simulink model "Copy_of_s_hover"  (Simulink 8.8)
settings: Solver=ode14x  StartTime=0.0  StopTime=inf  FixedStep=0.005  RelTol=1e-3  EnableMultiTasking=on
values from neighbouring files (symbols this model uses):
  b0_p = value    (= 0.1035)    [Copy_of_setup_lab_hover.m]
  b0_r = value    (= 0.1035)    [Copy_of_setup_lab_hover.m]
  b0_y = 0.0105    [Copy_of_setup_lab_hover.m]
  con = inv(con)    [Copy_of_setup_lab_hover.m]
  K_AMP = 3    [Copy_of_setup_lab_hover.m]    (also in setup_lab_hover.m; setup_lab_hover1.m)
  kd_p = 2 * wc_p    (= 23.3333333333)    [Copy_of_setup_lab_hover.m]
  kd_r = 2 * wc_r    (= 23.3333333333)    [Copy_of_setup_lab_hover.m]
  kd_y = 2 * wc_y    (= 8)    [Copy_of_setup_lab_hover.m]
  kp_p = wc_p ^ 2    (= 136.111111111)    [Copy_of_setup_lab_hover.m]
  kp_r = wc_r ^ 2    (= 136.111111111)    [Copy_of_setup_lab_hover.m]
  kp_y = wc_y ^ 2    (= 16)    [Copy_of_setup_lab_hover.m]
  VMAX_AMP = 24    [Copy_of_setup_lab_hover.m]    (also in setup_lab_hover.m; setup_lab_hover1.m)
  VMAX_DAC = 10    [Copy_of_setup_lab_hover.m]    (also in setup_lab_hover.m; setup_lab_hover1.m)
  w0_p = 35    [Copy_of_setup_lab_hover.m]
  w0_r = 35    [Copy_of_setup_lab_hover.m]
  w0_y = 28    [Copy_of_setup_lab_hover.m]
  wcf = 2 * pi * 20    (= 125.663706144)    [Copy_of_setup_lab_hover.m]    (also in setup_lab_hover.m; setup_lab_hover1.m)
  zetaf = 0.6    [Copy_of_setup_lab_hover.m]    (also in setup_lab_hover.m; setup_lab_hover1.m)
undefined symbols (not defined in the file or in its folder): A, B, C, D
libraries: simulink_extras x7, instrumentlib x2, aerolibanimutils x1
settings Model: LogicAnalyzerSignalOrdering=04bcc7a1-ed51-4d67-9ebe-09d7c85a2b61  SuppressorTable=22 serialization::archive 11 0 3 0 0 0 0 0  Creator=hpineros  LastModifiedBy=ronan  ExtModeTrigDuration=10000
settings SolverCC: PositivePriorityOrder=on
settings OptimizationCC: ExpressionDepthLimit=2147483647  InitFltsAndDblsToZero=on
settings DebuggingCC: SaveWithParameterizedLinksMsg=none  SolverPrmCheckMsg=warning
settings RTWCC: SystemTargetFile=quarc_windows.tlc  TemplateMakefile=quarc_default_tmf  Description=QuaRC Win32 Target
settings STFCustomTargetCC: TargetFcnLib=ansi_tfl_tmw.mat  TargetPreCompLibLocation=C:\PROGRA~3\QUARC\lib\2012b\windows\release  GeneratePreprocessorConditionals=Disable all  CPPClassGenCompliant=on  SystemTargetFile=quarc_windows.tlc
settings GRTTargetCC: TargetFcnLib=ansi_tfl_tmw.mat  TargetPreCompLibLocation=C:\PROGRA~3\QUARC\lib\2012b\windows\release  ParMdlRefBuildCompliant=off  CompOptLevelCompliant=off  ConcurrentExecutionCompliant=off  MatFileLogging=off  UseToolchainInfoCompliant=off  ExtMode=on  ExtModeMexFile=quarc_comm

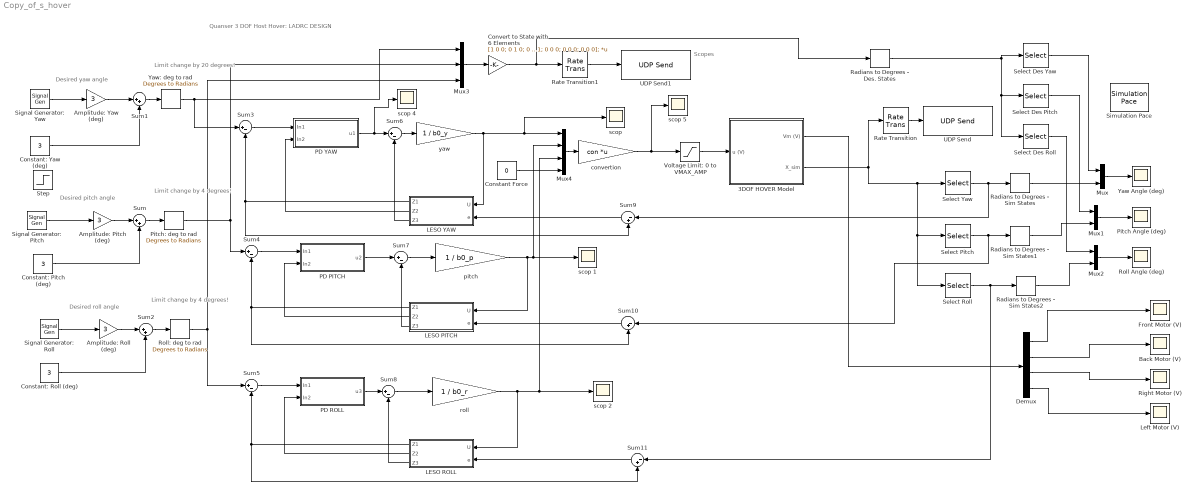
== system Copy_of_s_hover ==
  note: Quanser 3 DOF Host Hover:
      | LADRC DESIGN
  note: Scopes
  note: Limit change by
      | 4 degrees!
  note: Limit change by
      | 20 degrees!
  note: Limit change by
      | 4 degrees!
  note: Desired roll angle
  note: Desired pitch angle
  note: Desired yaw angle
  3DOF HOVER Model : Subsystem
  Amplitude: Pitch (deg) : Gain  Gain=3
  Amplitude: Roll (deg) : Gain  Gain=3
  Amplitude: Yaw (deg) : Gain  Gain=3
  Back Motor (V) : Scope
  Constant Force : Constant  Value=0
  Constant: Pitch (deg) : Constant  Value=3
  Constant: Roll (deg) : Constant  Value=3
  Constant: Yaw (deg) : Constant  Value=3
  Convert to State with 6 Elements : Gain  Gain=[1 0 0; 0 1 0; 0 0 1; 0 0 0; 0 0 0; 0 0 0];  Multiplication=Matrix(K*u)
  Demux : Demux
  Front Motor (V) : Scope
  LESO PITCH : Subsystem
  LESO ROLL : Subsystem
  LESO YAW : Subsystem
  Left Motor (V) : Scope
  Mux : Mux  Inputs=2
  Mux1 : Mux  Inputs=2
  Mux2 : Mux  Inputs=2
  Mux3 : Mux  Inputs=3
  Mux4 : Mux
  PD PITCH : Subsystem
  PD ROLL : Subsystem
  PD YAW : Subsystem
  Pitch Angle (deg) : Scope
  Pitch: deg to rad : simulink_extras/Transformations/Degrees to Radians
  Radians to Degrees - Des. States : simulink_extras/Transformations/Radians to Degrees
  Radians to Degrees - Sim States : simulink_extras/Transformations/Radians to Degrees
  Radians to Degrees - Sim States1 : simulink_extras/Transformations/Radians to Degrees
  Radians to Degrees - Sim States2 : simulink_extras/Transformations/Radians to Degrees
  Rate Transition : RateTransition  OutPortSampleTime=0.005
  Rate Transition1 : RateTransition  OutPortSampleTime=0.005
  Right Motor (V) : Scope
  Roll Angle (deg) : Scope
  Roll: deg to rad : simulink_extras/Transformations/Degrees to Radians
  Select Des Pitch : Selector  InputPortWidth=6  IndexOptions=Index vector (dialog)  Indices=2  OutputSizes=1
  Select Des Roll : Selector  InputPortWidth=6  IndexOptions=Index vector (dialog)  Indices=3  OutputSizes=1
  Select Des Yaw : Selector  InputPortWidth=6  IndexOptions=Index vector (dialog)  Indices=1  OutputSizes=1
  Select Pitch : Selector  InputPortWidth=6  IndexOptions=Index vector (dialog)  Indices=2  OutputSizes=1
  Select Roll : Selector  InputPortWidth=6  IndexOptions=Index vector (dialog)  Indices=3  OutputSizes=1
  Select Yaw : Selector  InputPortWidth=6  IndexOptions=Index vector (dialog)  Indices=1  OutputSizes=1
  Signal Generator: Pitch : SignalGenerator  WaveForm=square  Frequency=0.1
  Signal Generator: Roll : SignalGenerator  WaveForm=square  Frequency=0.08
  Signal Generator: Yaw : SignalGenerator  WaveForm=square  Frequency=0.04
  Simulation Pace : aerolibanimutils/Simulation Pace  SimulationPace=1  SleepMode=MATLAB Thread  OutputPaceError=off  SampleTime=0.01
  Step : Step  Time=0  SampleTime=0
  Sum : Sum  Inputs=|++
  Sum1 : Sum  Inputs=|++
  Sum10 : Sum  Inputs=|-+
  Sum11 : Sum  Inputs=|-+
  Sum2 : Sum  Inputs=|++
  Sum{3..8} (6 alike) : Sum  Inputs=|+-
  Sum9 : Sum  Inputs=|-+
  UDP Send : instrumentlib/UDP Send  Host=localhost  Port=9092  LocalPort=9091  EnableBlockingMode=on  ByteOrder=BigEndian
  UDP Send1 : instrumentlib/UDP Send  Host=localhost  Port=9094  LocalPort=9093  EnableBlockingMode=on  ByteOrder=BigEndian
  Voltage Limit: 0 to VMAX_AMP : Saturate  UpperLimit=VMAX_AMP  LowerLimit=0
  Yaw Angle (deg) : Scope
  Yaw: deg to rad : simulink_extras/Transformations/Degrees to Radians
  convertion : Gain  Gain=con  Multiplication=Matrix(K*u)  SaturateOnIntegerOverflow=on  OutDataTypeStr=Inherit: Same as input  ParamDataTypeStr=Inherit: Same as input
  pitch : Gain  Gain=1 / b0_p  SaturateOnIntegerOverflow=on  OutDataTypeStr=Inherit: Same as input  ParamDataTypeStr=Inherit: Same as input
  roll : Gain  Gain=1 / b0_r  SaturateOnIntegerOverflow=on  OutDataTypeStr=Inherit: Same as input  ParamDataTypeStr=Inherit: Same as input
  scop {,1..2,4..5} (5 alike) : Scope
  yaw : Gain  Gain=1 / b0_y  SaturateOnIntegerOverflow=on  OutDataTypeStr=Inherit: Same as input  ParamDataTypeStr=Inherit: Same as input
  wires:
  3DOF HOVER Model/1(Vm (V)) -> Demux/1
  Select Des Roll/1 -> Mux2/1
  Select Des Pitch/1 -> Mux1/1
  Select Des Yaw/1 -> Mux/1
  Radians to Degrees - Des. States/1 -> Select Des Yaw/1, Select Des Roll/1, Select Des Pitch/1
  Select Roll/1 -> Sum11/1, Radians to Degrees - Sim States2/1
  Select Pitch/1 -> Sum10/1, Radians to Degrees - Sim States1/1
  Select Yaw/1 -> Sum9/1, Radians to Degrees - Sim States/1
  Mux2/1 -> Roll Angle (deg)/1
  3DOF HOVER Model/2(X_sim) -> Select Yaw/1, Select Pitch/1, Select Roll/1, Rate Transition/1
  Mux1/1 -> Pitch Angle (deg)/1
  Mux/1 -> Yaw Angle (deg)/1
  Demux/1 -> Front Motor (V)/1
  Demux/2 -> Back Motor (V)/1
  Demux/3 -> Right Motor (V)/1
  Demux/4 -> Left Motor (V)/1
  Rate Transition/1 -> UDP Send/1
  Rate Transition1/1 -> UDP Send1/1
  Roll: deg to rad/1 -> Mux3/3, Sum5/1
  Pitch: deg to rad/1 -> Sum4/1, Mux3/2
  Yaw: deg to rad/1 -> Sum3/1, Mux3/1
  Sum2/1 -> Roll: deg to rad/1
  Amplitude: Roll (deg)/1 -> Sum2/1
  Constant: Roll (deg)/1 -> Sum2/2
  Sum/1 -> Pitch: deg to rad/1
  Amplitude: Pitch (deg)/1 -> Sum/1
  Constant: Pitch (deg)/1 -> Sum/2
  Sum1/1 -> Yaw: deg to rad/1
  Amplitude: Yaw (deg)/1 -> Sum1/1
  Constant: Yaw (deg)/1 -> Sum1/2
  Mux3/1 -> Convert to State with 6 Elements/1
  Convert to State with 6 Elements/1 -> Radians to Degrees - Des. States/1, Rate Transition1/1
  Sum3/1 -> PD YAW/1(In1)
  LESO YAW/1(Z1) -> Sum9/2, Sum3/2
  LESO PITCH/1(Z1) -> Sum10/2, Sum4/2
  LESO ROLL/1(Z1) -> Sum5/2, Sum11/2
  Sum5/1 -> PD ROLL/1(In1)
  Sum4/1 -> PD PITCH/1(In1)
  LESO YAW/2(Z2) -> PD YAW/2(In2)
  LESO PITCH/2(Z2) -> PD PITCH/2(In2)
  LESO ROLL/2(Z2) -> PD ROLL/2(In2)
  PD YAW/1(u1) -> scop 4/1, Sum6/1
  LESO YAW/3(Z3) -> Sum6/2
  PD PITCH/1(u2) -> Sum7/1
  LESO PITCH/3(Z3) -> Sum7/2
  PD ROLL/1(u3) -> Sum8/1
  LESO ROLL/3(Z3) -> Sum8/2
  Sum6/1 -> yaw/1
  yaw/1 -> LESO YAW/1(U), "scop "/1, Mux4/1
  Sum7/1 -> pitch/1
  Sum8/1 -> roll/1
  pitch/1 -> Mux4/2, scop 1/1, LESO PITCH/1(U)
  roll/1 -> scop 2/1, Mux4/3, LESO ROLL/1(U)
  Sum9/1 -> LESO YAW/2(e)
  Sum10/1 -> LESO PITCH/2(e)
  Sum11/1 -> LESO ROLL/2(e)
  convertion/1 -> Voltage Limit: 0 to VMAX_AMP/1, scop 5/1
  Mux4/1 -> convertion/1
  Constant Force/1 -> Mux4/4
  Voltage Limit: 0 to VMAX_AMP/1 -> 3DOF HOVER Model/1(u (V))
  Radians to Degrees - Sim States/1 -> Mux/2
  Radians to Degrees - Sim States1/1 -> Mux1/2
  Radians to Degrees - Sim States2/1 -> Mux2/2
  Signal Generator: Roll/1 -> Amplitude: Roll (deg)/1
  Signal Generator: Pitch/1 -> Amplitude: Pitch (deg)/1
  Signal Generator: Yaw/1 -> Amplitude: Yaw (deg)/1

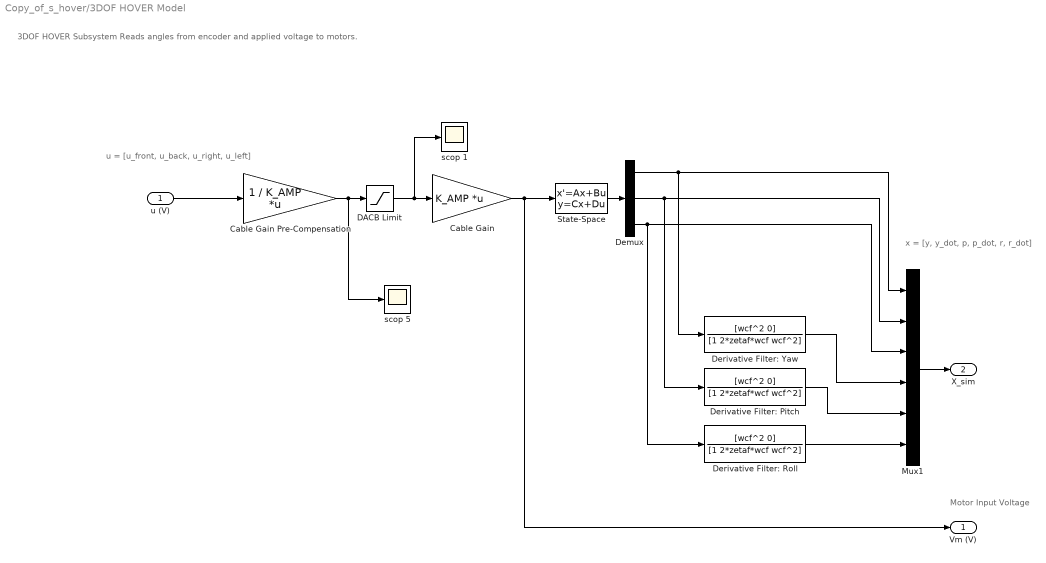
== system Copy_of_s_hover/3DOF HOVER Model ==
  note: 3DOF HOVER Subsystem
      | Reads angles from encoder and applied voltage to motors.
  note: Motor Input Voltage
  note: u = [u_front, u_back, u_right, u_left]
  note: x = [y, y_dot, p, p_dot, r, r_dot]
  u (V) : Inport
  Cable Gain : Gain  Gain=K_AMP  Multiplication=Matrix(K*u)  SaturateOnIntegerOverflow=on  OutDataTypeStr=Inherit: Same as input  ParamDataTypeStr=Inherit: Same as input
  Cable Gain Pre-Compensation : Gain  Gain=1 / K_AMP  Multiplication=Matrix(K*u)  SaturateOnIntegerOverflow=on  OutDataTypeStr=Inherit: Same as input  ParamDataTypeStr=Inherit: Same as input
  DACB Limit : Saturate  UpperLimit=VMAX_DAC  LowerLimit=-VMAX_DAC
  Demux : Demux  Outputs=3
  Derivative Filter: Pitch : TransferFcn  Numerator=[wcf^2 0]  Denominator=[1 2*zetaf*wcf wcf^2]
  Derivative Filter: Roll : TransferFcn  Numerator=[wcf^2 0]  Denominator=[1 2*zetaf*wcf wcf^2]
  Derivative Filter: Yaw : TransferFcn  Numerator=[wcf^2 0]  Denominator=[1 2*zetaf*wcf wcf^2]
  Mux1 : Mux  Inputs=6
  State-Space : StateSpace  A=A  B=B  C=C  D=D  X0=0
  scop 1 : Scope
  scop 5 : Scope
  Vm (V) : Outport
  X_sim : Outport  Port=2
  wires:
  Demux/3 -> Derivative Filter: Roll/1, Mux1/3
  Demux/2 -> Derivative Filter: Pitch/1, Mux1/2
  Derivative Filter: Roll/1 -> Mux1/6
  Derivative Filter: Pitch/1 -> Mux1/5
  Derivative Filter: Yaw/1 -> Mux1/4
  Demux/1 -> Derivative Filter: Yaw/1, Mux1/1
  State-Space/1 -> Demux/1
  Mux1/1 -> X_sim/1
  Cable Gain/1 -> State-Space/1, Vm (V)/1
  DACB Limit/1 -> scop 1/1, Cable Gain/1
  Cable Gain Pre-Compensation/1 -> scop 5/1, DACB Limit/1
  u (V)/1 -> Cable Gain Pre-Compensation/1

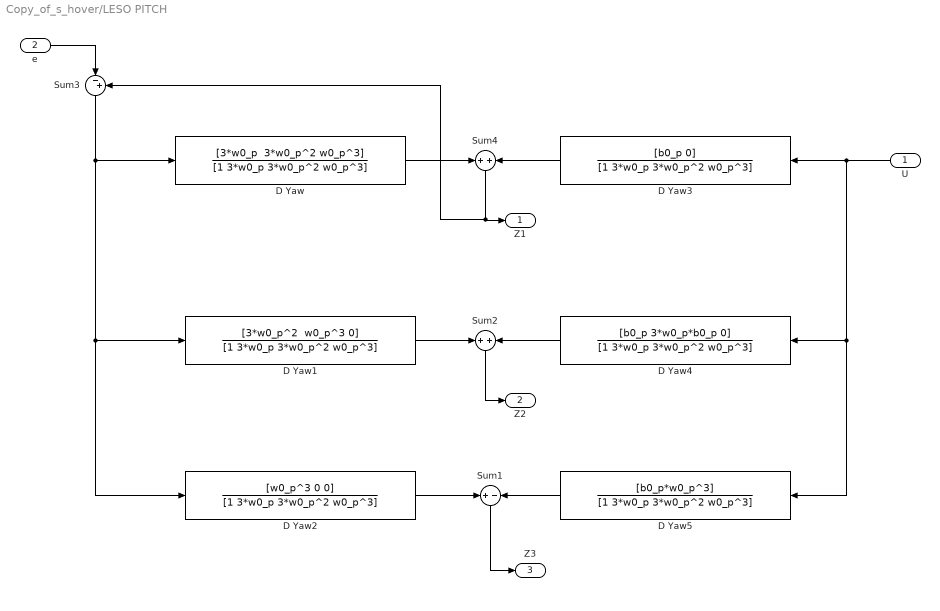
== system Copy_of_s_hover/LESO PITCH ==
  U : Inport
  e : Inport  Port=2
  D Yaw : TransferFcn  Numerator="[3*w0_p  3*w0_p^2 w0_p^3]"  Denominator=[1 3*w0_p 3*w0_p^2 w0_p^3]
  D Yaw1 : TransferFcn  Numerator="[3*w0_p^2  w0_p^3 0]"  Denominator=[1 3*w0_p 3*w0_p^2 w0_p^3]
  D Yaw2 : TransferFcn  Numerator=[w0_p^3 0 0]  Denominator=[1 3*w0_p 3*w0_p^2 w0_p^3]
  D Yaw3 : TransferFcn  Numerator=[b0_p 0]  Denominator=[1 3*w0_p 3*w0_p^2 w0_p^3]
  D Yaw4 : TransferFcn  Numerator=[b0_p 3*w0_p*b0_p 0]  Denominator=[1 3*w0_p 3*w0_p^2 w0_p^3]
  D Yaw5 : TransferFcn  Numerator=[b0_p*w0_p^3]  Denominator=[1 3*w0_p 3*w0_p^2 w0_p^3]
  Sum1 : Sum  Inputs=+|-
  Sum2 : Sum  Inputs=+|+
  Sum3 : Sum  Inputs=|-+
  Sum4 : Sum  Inputs=+|+
  Z1 : Outport
  Z2 : Outport  Port=2
  Z3 : Outport  Port=3
  wires:
  e/1 -> Sum3/1
  Sum3/1 -> D Yaw2/1, D Yaw1/1, D Yaw/1
  U/1 -> D Yaw5/1, D Yaw4/1, D Yaw3/1
  D Yaw2/1 -> Sum1/1
  D Yaw5/1 -> Sum1/2
  Sum1/1 -> Z3/1
  D Yaw1/1 -> Sum2/1
  D Yaw4/1 -> Sum2/2
  Sum2/1 -> Z2/1
  D Yaw/1 -> Sum4/1
  D Yaw3/1 -> Sum4/2
  Sum4/1 -> Sum3/2, Z1/1

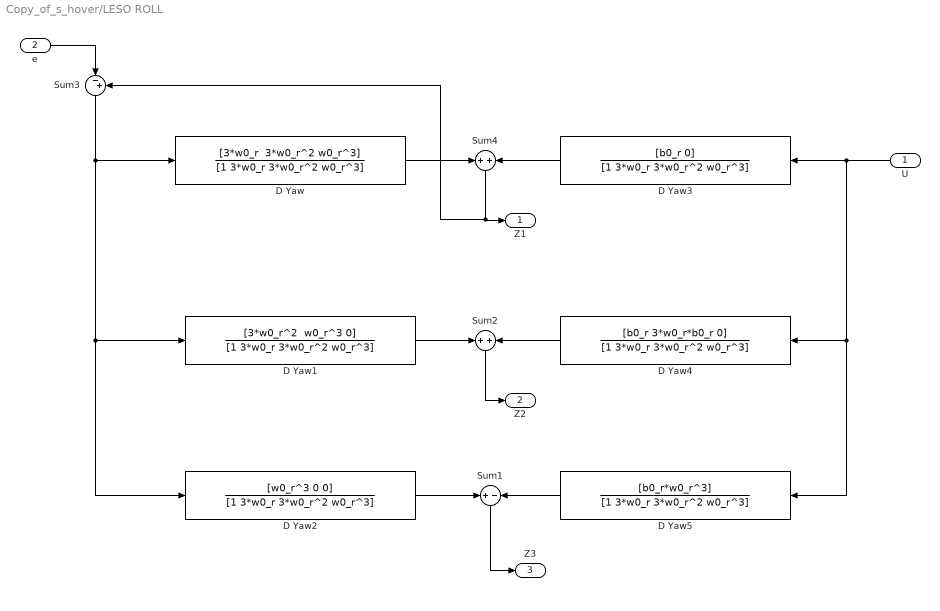
== system Copy_of_s_hover/LESO ROLL ==
  U : Inport
  e : Inport  Port=2
  D Yaw : TransferFcn  Numerator="[3*w0_r  3*w0_r^2 w0_r^3]"  Denominator=[1 3*w0_r 3*w0_r^2 w0_r^3]
  D Yaw1 : TransferFcn  Numerator="[3*w0_r^2  w0_r^3 0]"  Denominator=[1 3*w0_r 3*w0_r^2 w0_r^3]
  D Yaw2 : TransferFcn  Numerator=[w0_r^3 0 0]  Denominator=[1 3*w0_r 3*w0_r^2 w0_r^3]
  D Yaw3 : TransferFcn  Numerator=[b0_r 0]  Denominator=[1 3*w0_r 3*w0_r^2 w0_r^3]
  D Yaw4 : TransferFcn  Numerator=[b0_r 3*w0_r*b0_r 0]  Denominator=[1 3*w0_r 3*w0_r^2 w0_r^3]
  D Yaw5 : TransferFcn  Numerator=[b0_r*w0_r^3]  Denominator=[1 3*w0_r 3*w0_r^2 w0_r^3]
  Sum1 : Sum  Inputs=+|-
  Sum2 : Sum  Inputs=+|+
  Sum3 : Sum  Inputs=|-+
  Sum4 : Sum  Inputs=+|+
  Z1 : Outport
  Z2 : Outport  Port=2
  Z3 : Outport  Port=3
  wires:
  e/1 -> Sum3/1
  Sum3/1 -> D Yaw2/1, D Yaw1/1, D Yaw/1
  U/1 -> D Yaw5/1, D Yaw4/1, D Yaw3/1
  D Yaw2/1 -> Sum1/1
  D Yaw5/1 -> Sum1/2
  Sum1/1 -> Z3/1
  D Yaw1/1 -> Sum2/1
  D Yaw4/1 -> Sum2/2
  Sum2/1 -> Z2/1
  D Yaw/1 -> Sum4/1
  D Yaw3/1 -> Sum4/2
  Sum4/1 -> Sum3/2, Z1/1

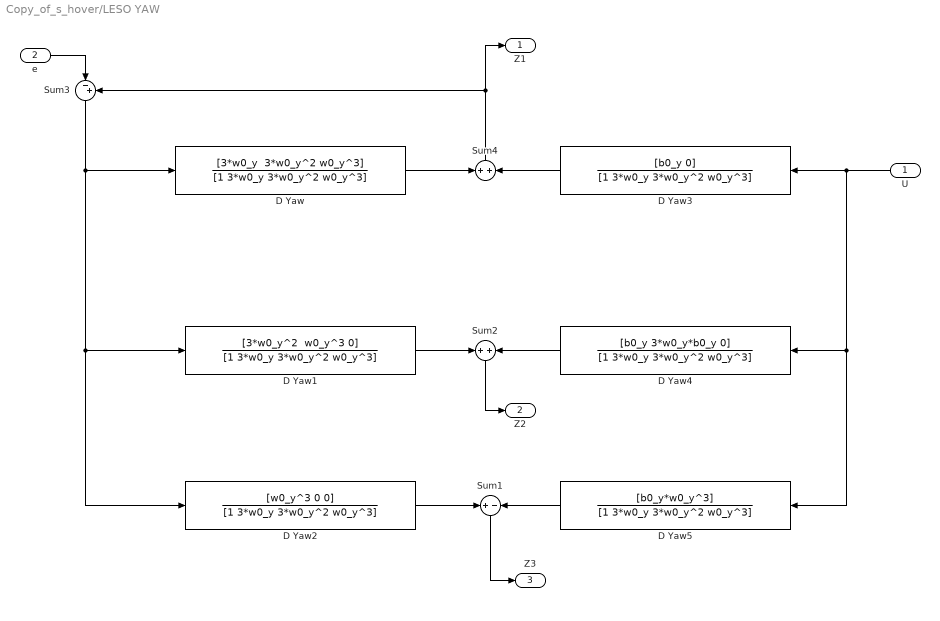
== system Copy_of_s_hover/LESO YAW ==
  U : Inport
  e : Inport  Port=2
  D Yaw : TransferFcn  Numerator="[3*w0_y  3*w0_y^2 w0_y^3]"  Denominator=[1 3*w0_y 3*w0_y^2 w0_y^3]
  D Yaw1 : TransferFcn  Numerator="[3*w0_y^2  w0_y^3 0]"  Denominator=[1 3*w0_y 3*w0_y^2 w0_y^3]
  D Yaw2 : TransferFcn  Numerator=[w0_y^3 0 0]  Denominator=[1 3*w0_y 3*w0_y^2 w0_y^3]
  D Yaw3 : TransferFcn  Numerator=[b0_y 0]  Denominator=[1 3*w0_y 3*w0_y^2 w0_y^3]
  D Yaw4 : TransferFcn  Numerator=[b0_y 3*w0_y*b0_y 0]  Denominator=[1 3*w0_y 3*w0_y^2 w0_y^3]
  D Yaw5 : TransferFcn  Numerator=[b0_y*w0_y^3]  Denominator=[1 3*w0_y 3*w0_y^2 w0_y^3]
  Sum1 : Sum  Inputs=+|-
  Sum2 : Sum  Inputs=+|+
  Sum3 : Sum  Inputs=|-+
  Sum4 : Sum  Inputs=+|+
  Z1 : Outport
  Z2 : Outport  Port=2
  Z3 : Outport  Port=3
  wires:
  U/1 -> D Yaw5/1, D Yaw4/1, D Yaw3/1
  D Yaw2/1 -> Sum1/1
  D Yaw5/1 -> Sum1/2
  Sum1/1 -> Z3/1
  D Yaw1/1 -> Sum2/1
  D Yaw4/1 -> Sum2/2
  Sum2/1 -> Z2/1
  D Yaw/1 -> Sum4/1
  D Yaw3/1 -> Sum4/2
  Sum4/1 -> Z1/1, Sum3/2
  e/1 -> Sum3/1
  Sum3/1 -> D Yaw1/1, D Yaw2/1, D Yaw/1

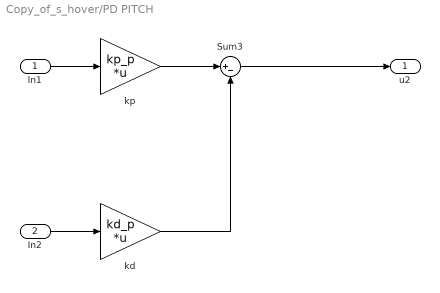
== system Copy_of_s_hover/PD PITCH ==
  In1 : Inport
  In2 : Inport  Port=2
  Sum3 : Sum  Inputs=|+-
  kd : Gain  Gain=kd_p  Multiplication=Matrix(K*u)  SaturateOnIntegerOverflow=on  OutDataTypeStr=Inherit: Same as input  ParamDataTypeStr=Inherit: Same as input
  kp : Gain  Gain=kp_p  Multiplication=Matrix(K*u)  SaturateOnIntegerOverflow=on  OutDataTypeStr=Inherit: Same as input  ParamDataTypeStr=Inherit: Same as input
  u2 : Outport
  wires:
  In1/1 -> kp/1
  In2/1 -> kd/1
  kp/1 -> Sum3/1
  kd/1 -> Sum3/2
  Sum3/1 -> u2/1

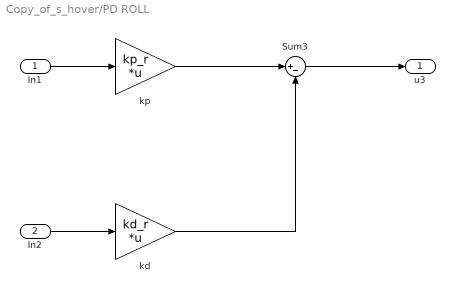
== system Copy_of_s_hover/PD ROLL ==
  In1 : Inport
  In2 : Inport  Port=2
  Sum3 : Sum  Inputs=|+-
  kd : Gain  Gain=kd_r  Multiplication=Matrix(K*u)  SaturateOnIntegerOverflow=on  OutDataTypeStr=Inherit: Same as input  ParamDataTypeStr=Inherit: Same as input
  "kp " : Gain  Gain=kp_r  Multiplication=Matrix(K*u)  SaturateOnIntegerOverflow=on  OutDataTypeStr=Inherit: Same as input  ParamDataTypeStr=Inherit: Same as input
  u3 : Outport
  wires:
  In1/1 -> "kp "/1
  In2/1 -> kd/1
  "kp "/1 -> Sum3/1
  kd/1 -> Sum3/2
  Sum3/1 -> u3/1

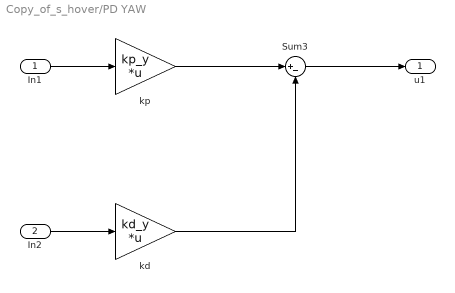
== system Copy_of_s_hover/PD YAW ==
  In1 : Inport
  In2 : Inport  Port=2
  Sum3 : Sum  Inputs=|+-
  kd : Gain  Gain=kd_y  Multiplication=Matrix(K*u)  SaturateOnIntegerOverflow=on  OutDataTypeStr=Inherit: Same as input  ParamDataTypeStr=Inherit: Same as input
  kp : Gain  Gain=kp_y  Multiplication=Matrix(K*u)  SaturateOnIntegerOverflow=on  OutDataTypeStr=Inherit: Same as input  ParamDataTypeStr=Inherit: Same as input
  u1 : Outport
  wires:
  In1/1 -> kp/1
  In2/1 -> kd/1
  kp/1 -> Sum3/1
  kd/1 -> Sum3/2
  Sum3/1 -> u1/1
